simulink model "VehicleSilSimulation"  (R2026a)
settings: configuration reference "standardSILConfigurationParams" (kept outside this file)
StopFcn:
  | fid = fopen('C:\Users\Edison Altamirano\SITLV2\AnelloSummer\optimAeroPX4SIL\HILDiagnostics\logs\session_gtfix1\matlab_error_capture.txt','a'); fprintf(fid, '--- StopFcn fired at %s ---\n', datestr(now)); [m,i] = lasterr(); fprintf(fid, 'lasterr: %s (id: %s)\n', m, i); try; le = lasterror(); fprintf(fid, 'stack:\n'); for k=1:numel(le.stack); fprintf(fid, '  %s line %d\n', le.stack(k).name, le.stack(k).line); end; catch; end; fclose(fid);
values from neighbouring files (symbols this model uses):
  CONTROLLER_RUNTIME = 1    [initVehicleSIL.m]
  stepSize_s = 0.004    [initVehicleSIL.m]
  vehicleParams = evalin('base', 'vehicleParams')    [testVehicleSIL.m]
undefined symbols (not defined in the file or in its folder): actuatorDelay_s, controllerArmed, EngineCommandBus, gpsFreq, heartbeatFreq, opts, Payload, plantSampleTime_s, referenceLatitude_deg, referenceLongitude_deg, SampleTime, ServosCommandBus
libraries: uavmavlinklib x8, simulink x8, instrumentlib x6, flightGearInterfaceLibrary x6, aerolibfltsims x3, sharedtransform x3, px4MAVLinkBridgelib x2, aerolibanimutils x1, hdlsllib x1, dspnetwork x1, robotcorelib x1, uavutilslib x1
(part 1 of 3)
settings Model: SimulationMode=accelerator  Creator=GTAR  LastModifiedBy=Edison Altamirano
settings ConfigSetRef: SourceName=standardSILConfigurationParams  SourceLocation=Base Workspace

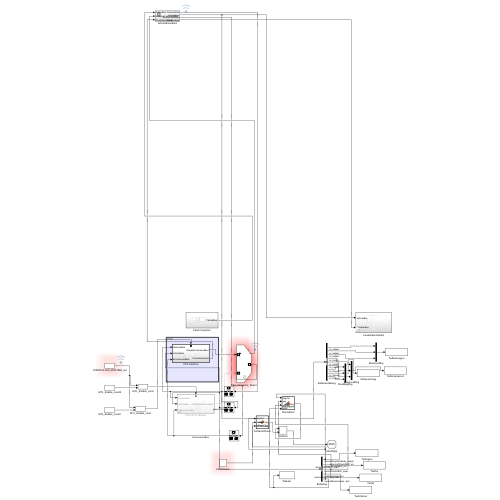
[thumbnail: Simulink's stored preview of the top-level diagram]
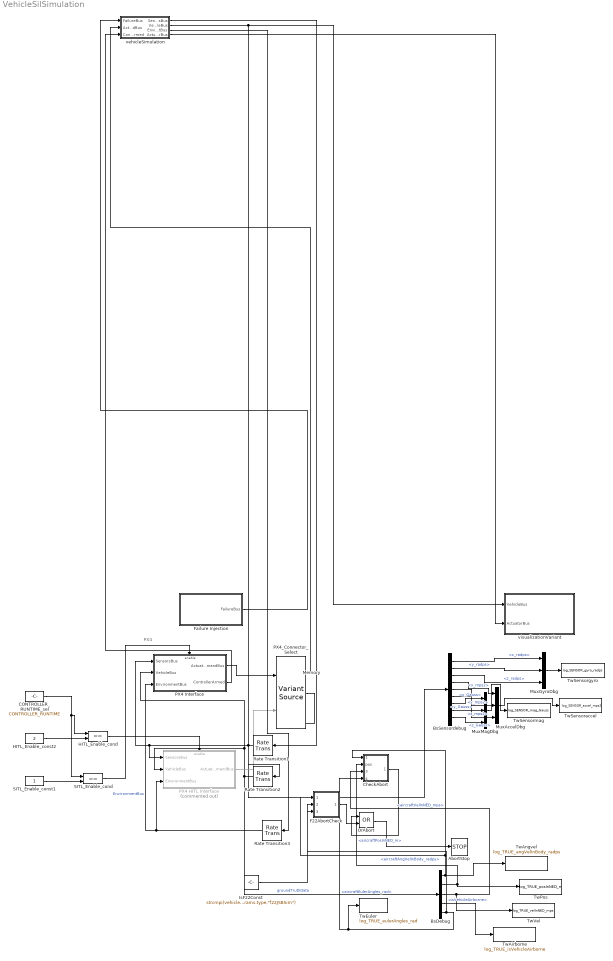
== system VehicleSilSimulation ==
  note: PX4
  AbortStop : Stop
  BsDebug : BusSelector  OutputSignals=signal2.aircraftAngVelInBody_radps,signal2.aircraftPosInNED_m,signal2.aircraftVelInNED_mps,signal1.isVehicleAirborne,signal2.aircraftEulerAngles_rad
  BsSensordebug : BusSelector  OutputSignals=INSSensorBus.GyroSensorBus.x_radps,INSSensorBus.GyroSensorBus.y_radps,INSSensorBus.GyroSensorBus.z_radps,INSSensorBus.AccelSensorBus.x_mps2,INSSensorBus.AccelSensorBus.y_mps2,INSSensorBus.AccelSensorBus.z_mps2,INSSensorBus.MagSensorBus.x_Gauss,INSSensorBus.MagSensorBus.y_Gauss,INSSensorBus.MagSensorBus.z_Gauss
  CONTROLLER_RUNTIME_sel : Constant  Value=CONTROLLER_RUNTIME
  CheckAbort : MATLAB Function  TreatAsAtomicUnit=on
  F22AbortCheck : MATLAB Function  TreatAsAtomicUnit=on
  Failure Injection : Subsystem
  HITL_Enable_cond : RelationalOperator  Operator===  OutDataTypeStr=boolean  RndMeth=Simplest  InputSameDT=off
  HITL_Enable_const2 : Constant  Value=2
  IsF22Const : Constant  Value="strcmpi(vehicleParams.type,\"f22JSBSim\")"
  Memory : Memory
  MuxAccelDbg : Mux  Inputs=3
  MuxGyroDbg : Mux  Inputs=3
  MuxMagDbg : Mux  Inputs=3
  OrAbort : Logic  Operator=OR
  PX4 HITL Interface : Subsystem  Commented=on
  PX4 Interface : Subsystem  VariantControl="strcmpi(vehicleParams.type, \"F-16\") & strcmpi(vehicleParams.controllerType, \"PX4\")"
  PX4_Connector_Select : VariantSource  VariantControls={CONTROLLER_RUNTIME == 1, CONTROLLER_RUNTIME == 2}
  Rate Transition1 : RateTransition
  Rate Transition2 : RateTransition
  Rate Transition3 : RateTransition
  SITL_Enable_cond : RelationalOperator  Operator===  OutDataTypeStr=boolean  RndMeth=Simplest  InputSameDT=off
  SITL_Enable_const1 : Constant
  TwAirborne : ToWorkspace  VariableName=log_TRUE_isVehicleAirborne  SaveFormat=Structure With Time  SampleTime=-1
  TwAngvel : ToWorkspace  VariableName=log_TRUE_angVelInBody_radps  SaveFormat=Structure With Time  SampleTime=-1
  TwEuler : ToWorkspace  VariableName=log_TRUE_eulerAngles_rad  SaveFormat=Timeseries  SampleTime=-1
  TwPos : ToWorkspace  VariableName=log_TRUE_posInNED_m  SaveFormat=Structure With Time  SampleTime=-1
  TwSensoraccel : ToWorkspace  VariableName=log_SENSOR_accel_mps2  SaveFormat=Structure With Time  SampleTime=-1
  TwSensorgyro : ToWorkspace  VariableName=log_SENSOR_gyro_radps  SaveFormat=Structure With Time  SampleTime=-1
  TwSensormag : ToWorkspace  VariableName=log_SENSOR_mag_Gauss  SaveFormat=Structure With Time  SampleTime=-1
  TwVel : ToWorkspace  VariableName=log_TRUE_velInNED_mps  SaveFormat=Structure With Time  SampleTime=-1
  vehicleSimulation : Subsystem
  visualizationVariant : Subsystem  Variant=on  EmptyChoice=on
  wires:
  Rate Transition1/1 -> PX4 Interface/1(SensorsBus), PX4 HITL Interface/1(SensorsBus), BsSensordebug/1
  Rate Transition2/1 -> PX4 HITL Interface/2(VehicleBus), PX4 Interface/2(VehicleBus), BsDebug/1  "groundTruthData"
  Rate Transition3/1 -> PX4 Interface/3(EnvironmentBus), PX4 HITL Interface/3(EnvironmentBus)  "EnvironmentBus"
  CONTROLLER_RUNTIME_sel/1 -> HITL_Enable_cond/1, SITL_Enable_cond/1
  HITL_Enable_const2/1 -> HITL_Enable_cond/2
  HITL_Enable_cond/1 -> PX4 HITL Interface/Enable
  SITL_Enable_const1/1 -> SITL_Enable_cond/2
  SITL_Enable_cond/1 -> PX4 Interface/Enable
  PX4 Interface/1(ActuatorCommandBus) -> PX4_Connector_Select/1
  PX4 HITL Interface/1(ActuatorCommandBus) -> PX4_Connector_Select/2
  PX4_Connector_Select/1 -> Memory/1
  BsDebug/1 -> F22AbortCheck/1(angVel), CheckAbort/1(angVel), TwAngvel/1  "<aircraftAngVelInBody_radps>"
  BsDebug/2 -> TwPos/1, CheckAbort/2(pos)  "<aircraftPosInNED_m>"
  BsDebug/3 -> TwVel/1, CheckAbort/3(velNED)  "<aircraftVelInNED_mps>"
  BsDebug/4 -> TwAirborne/1  "<isVehicleAirborne>"
  BsSensordebug/1 -> MuxGyroDbg/1  "<x_radps>"
  BsSensordebug/2 -> MuxGyroDbg/2  "<y_radps>"
  BsSensordebug/3 -> MuxGyroDbg/3  "<z_radps>"
  BsSensordebug/4 -> MuxAccelDbg/1  "<x_mps2>"
  BsSensordebug/5 -> MuxAccelDbg/2  "<y_mps2>"
  BsSensordebug/6 -> MuxAccelDbg/3  "<z_mps2>"
  MuxGyroDbg/1 -> TwSensorgyro/1
  MuxAccelDbg/1 -> TwSensoraccel/1
  BsDebug/5 -> TwEuler/1, CheckAbort/4(euler), F22AbortCheck/2(euler)  "<aircraftEulerAngles_rad>"
  BsSensordebug/7 -> MuxMagDbg/1  "<x_Gauss>"
  BsSensordebug/8 -> MuxMagDbg/2  "<y_Gauss>"
  BsSensordebug/9 -> MuxMagDbg/3  "<z_Gauss>"
  MuxMagDbg/1 -> TwSensormag/1
  CheckAbort/1(abortFlag) -> OrAbort/1
  F22AbortCheck/1(abortFlag) -> OrAbort/2
  OrAbort/1 -> AbortStop/1
  IsF22Const/1 -> F22AbortCheck/3(isF22Active)
  vehicleSimulation/1(SensorsBus) -> Rate Transition1/1
  vehicleSimulation/2(VehicleBus) -> Rate Transition2/1, visualizationVariant/1(VehicleBus)
  vehicleSimulation/3(EnvironmentBus) -> Rate Transition3/1
  vehicleSimulation/4(ActuatorBus) -> visualizationVariant/2(ActuatorBus)
  Failure Injection/1(FailureBus) -> vehicleSimulation/1(FailureBus)
  Memory/1 -> vehicleSimulation/2(ActuatorCommandBus)
  PX4 Interface/2(ControllerArmed) -> vehicleSimulation/3(ControllerArmed)

== system VehicleSilSimulation/Failure Injection ==
  Constant : Constant  Value=vehicleParams.failureType
  PilotJoystick : aerolibanimutils/Pilot Joystick  JoystickID=None  OutputConfiguration=AllOutputs  SampleTime=stepSize_s
      settings: LibrarySourceBlock=aerolibanimutils/Pilot Joystick All
  Variant Model : Subsystem  Variant=on
  FailureBus : Outport
  wires:
  PilotJoystick/2 -> Variant Model/2(buttons)
  Variant Model/1(FailureBus) -> FailureBus/1
  PilotJoystick/3 -> Variant Model/3(POV)
  PilotJoystick/1 -> Variant Model/1(analog)
  Constant/1 -> Variant Model/4(failureType)

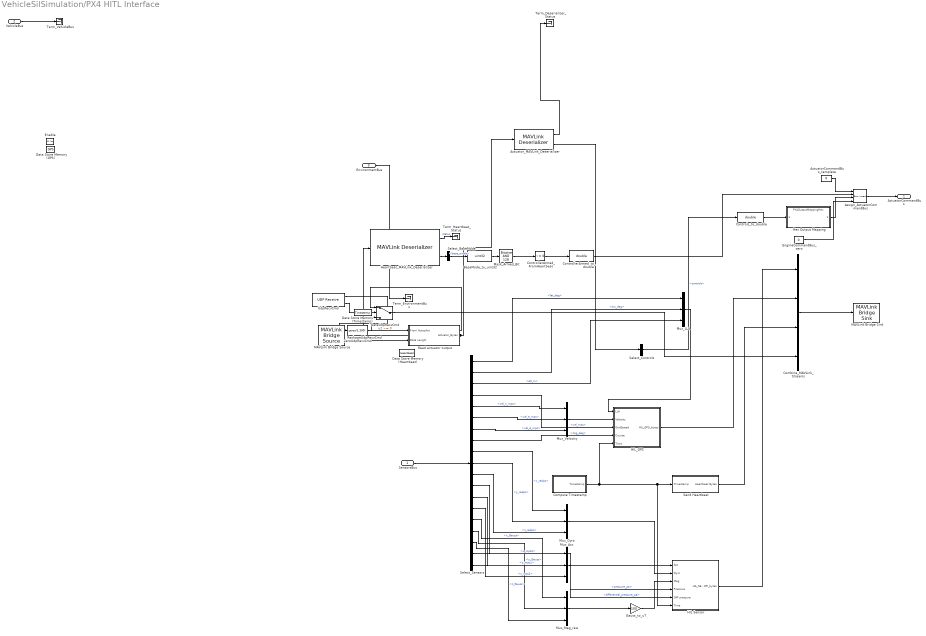
== system VehicleSilSimulation/PX4 HITL Interface ==
  SensorsBus : Inport  OutDataTypeStr=Bus: SensorsBus
  VehicleBus : Inport  Port=2  OutDataTypeStr=Bus: VehicleBus
  EnvironmentBus : Inport  Port=3  OutDataTypeStr=Bus: EnvironmentBus
  Enable : EnablePort  PropagateVarSize=During execution
  ActuatorCommandBus_template : Constant  Value=0  OutDataTypeStr=Bus: ActuatorCommandBus
  Actuator_MAVLink_Deserializer : uavmavlinklib/MAVLink Deserializer  dialectSource=Select from standard MAVLink dialects  dialect=common.xml  dialectCustom=common.xml  version=2  messageType=HIL_ACTUATOR_CONTROLS  inputDataLength=off  SystemIDFilter=off  systemID=1  ComponentIDFilter=off  componentID=1  queueMsg=off  queueMsgSize=50  dropNum=off
  Assign_ActuatorCommandBus : BusAssignment  AssignedSignals=controllerArmed,ServosCommandBus,EngineCommandBus
  BaseMode_to_uint32 : DataTypeConversion  OutDataTypeStr=uint32
  Combine_MAVLink_Streams : Mux
  Compute Timestamp : Subsystem  Priority=1
  ControllerArmed_FromHeartbeat : hdlsllib/Logic and Bit Operations/Compare To Zero  relop=~=  OutDataTypeStr=uint8
  ControllerArmed_to_double : DataTypeConversion  OutDataTypeStr=double
  Controls_to_double : DataTypeConversion  OutDataTypeStr=double  SaturateOnIntegerOverflow=off  RndMeth=Floor
  Data Store Memory (GPS) : DataStoreMemory  DataStoreName=GPS  WriteAfterWriteMsg=warning  ShowAdditionalParam=off
  Data Store Memory (Heartbeat) : DataStoreMemory  DataStoreName=Heartbeat  WriteAfterWriteMsg=warning  ShowAdditionalParam=off
  Data Store Memory (Timestamp) : DataStoreMemory  DataStoreName=Timestamp  WriteAfterWriteMsg=warning  ShowAdditionalParam=off
  EngineCommandBus_zero : Constant  Value=0  OutDataTypeStr=Bus: EngineCommandBus
  GateUdpRecvCmd : Switch  Criteria=u2 ~= 0  SaturateOnIntegerOverflow=off  InputSameDT=off
  Gauss_to_uT : Gain  Gain=100
  HIL Sensor : Subsystem  Priority=2
  HIL_GPS : Subsystem  Priority=3
  Heartbeat_MAVLink_Deserializer : uavmavlinklib/MAVLink Deserializer  dialectSource=Select from standard MAVLink dialects  dialect=common.xml  dialectCustom=common.xml  version=2  messageType=HEARTBEAT  inputDataLength=off  SystemIDFilter=off  systemID=1  ComponentIDFilter=off  componentID=1  queueMsg=off  queueMsgSize=50  dropNum=off
  Hex Output Mapping : ModelReference  ModelNameDialog=PX4OutputMappingHex.slx  SimulationMode=Normal  ModelReferenceVersion=1.15
  MAVLink Bridge Sink : px4MAVLinkBridgelib/MAVLink Bridge Sink  PixhawkSerialPorttemp=Specify manually  PixhawkSerialPortManually=COM4  FieldTable={'UDP', '127.0.0.1', '14550'}
  MAVLink Bridge Source : px4MAVLinkBridgelib/MAVLink Bridge Source  PixhawkSerialPorttemp=Specify manually  PixhawkSerialPortManually=COM4  dataLength=1024  FieldTable={'UDP', '127.0.0.1', '14550'}  SampleTime=SampleTime
  Mask_Armed_Bit : simulink/Logic and Bit Operations/Bitwise Operator  logicop=AND  UseBitMask=on  BitMask=128  BitMaskRealWorld=Stored Integer
      settings: LibrarySourceBlock=|
      | hdlsllib/Logic and Bit
      | Operations/Bitwise
      | Operator
  Mux_Acc : Mux  Inputs=3
  Mux_Gyro : Mux  Inputs=3
  Mux_LLA : Mux  Inputs=3
  Mux_Mag_raw : Mux  Inputs=3
  Mux_Velocity : Mux  Inputs=3
  Read actuator output : Subsystem
  ReshapeUdpRecvCmd : Reshape
  Select_BaseMode : BusSelector  OutputSignals=Payload.base_mode
  Select_Controls : BusSelector  OutputSignals=Payload.controls
  Select_Sensors : BusSelector  OutputSignals=GPSSensorBus.lat_deg,GPSSensorBus.lon_deg,GPSSensorBus.alt_m,GPSSensorBus.vel_mps,GPSSensorBus.vel_n_mps,GPSSensorBus.vel_e_mps,GPSSensorBus.vel_d_mps,GPSSensorBus.cog_deg,INSSensorBus.GyroSensorBus.x_radps,INSSensorBus.GyroSensorBus.y_radps,INSSensorBus.GyroSensorBus.z_radps,INSSensorBus.AccelSensorBus.x_mps2,INSSensorBus.AccelSensorBus.y_mps2,INSSensorBus.AccelSensorBus.z_mps2,INSSensorBus.MagSensorBus.x_Gauss,INSSensorBus.MagSensorBus.y_Gauss,INSSensorBus.MagSensorBus.z_Gauss,ADCSensorBus.BaroSensorBus.pressure_pa,ADCSensorBus.DiffPressureSensorBus.differential_pressure_pa
  Send Heartbeat : Subsystem  Priority=4
  Term_Deserializer_Status : Terminator
  Term_EnvironmentBus : Terminator
  Term_Heartbeat_Status : Terminator
  Term_VehicleBus : Terminator
  UdpRecvCmd : dspnetwork/UDP Receive  localURL='0.0.0.0'  localPort=14541  remoteURL='0.0.0.0'  remotePort=-1  recvBufferSize=8192  dims=300  signalDatatype=uint8  isComplex=off  isVarSize=off  showBlockingTime=off  blockingTime=0  sampletime=SampleTime  blockPlatform=[]
      settings: LibrarySourceBlock=dspsrcs4/UDP Receive
  ZeroUdpRecvCmd : Constant  Value=zeros(1,300)  OutDataTypeStr=uint8
  ActuatorCommandBus : Outport  OutDataTypeStr=Bus: ActuatorCommandBus
  wires:
  Select_Sensors/18 -> HIL Sensor/4(Pressure)  "<pressure_pa>"
  Select_Sensors/1 -> Mux_LLA/1  "<lat_deg>"
  HIL_GPS/1(HIL_GPS_bytes) -> Combine_MAVLink_Streams/2
  Actuator_MAVLink_Deserializer/1 -> Term_Deserializer_Status/1
  VehicleBus/1 -> Term_VehicleBus/1
  MAVLink Bridge Source/2 -> Read actuator output/2(Data Length)
  Read actuator output/1(Actuator_Bytes) -> Actuator_MAVLink_Deserializer/1, Heartbeat_MAVLink_Deserializer/1
  Mux_Mag_raw/1 -> Gauss_to_uT/1
  SensorsBus/1 -> Select_Sensors/1
  EnvironmentBus/1 -> Term_EnvironmentBus/1
  MAVLink Bridge Source/1 -> Read actuator output/1(From Autopilot)
  Select_Sensors/2 -> Mux_LLA/2  "<lon_deg>"
  Mux_Acc/1 -> HIL Sensor/1(Acc)
  Select_Sensors/3 -> Mux_LLA/3  "<alt_m>"
  Mux_Gyro/1 -> HIL Sensor/2(Gyro)
  Actuator_MAVLink_Deserializer/2 -> Select_Controls/1
  Select_Sensors/4 -> HIL_GPS/3(GndSpeed)  "<vel_mps>"
  Select_Sensors/5 -> Mux_Velocity/1  "<vel_n_mps>"
  Select_Sensors/11 -> Mux_Gyro/3  "<z_radps>"
  Select_Sensors/6 -> Mux_Velocity/2  "<vel_e_mps>"
  Select_Sensors/7 -> Mux_Velocity/3  "<vel_d_mps>"
  Mux_Velocity/1 -> HIL_GPS/2(Velocity)
  Select_Sensors/8 -> HIL_GPS/4(Course)  "<cog_deg>"
  HIL Sensor/1(HIL_SENSOR_bytes) -> Combine_MAVLink_Streams/1
  Select_Sensors/9 -> Mux_Gyro/1  "<x_radps>"
  ActuatorCommandBus_template/1 -> Assign_ActuatorCommandBus/1
  Select_Sensors/10 -> Mux_Gyro/2  "<y_radps>"
  Select_Sensors/12 -> Mux_Acc/1  "<x_mps2>"
  Select_Sensors/13 -> Mux_Acc/2  "<y_mps2>"
  Select_Sensors/14 -> Mux_Acc/3  "<z_mps2>"
  Select_Sensors/15 -> Mux_Mag_raw/1  "<x_Gauss>"
  Select_Sensors/16 -> Mux_Mag_raw/2  "<y_Gauss>"
  Select_Sensors/17 -> Mux_Mag_raw/3  "<z_Gauss>"
  Select_Sensors/19 -> HIL Sensor/5(Diff pressure)  "<differential_pressure_pa>"
  Mux_LLA/1 -> HIL_GPS/1(LLA)
  Compute Timestamp/1(Timestamp) -> HIL Sensor/6(Time), Send Heartbeat/1(Timestamp), HIL_GPS/5(Time)
  Controls_to_double/1 -> Hex Output Mapping/1
  Select_Controls/1 -> Controls_to_double/1  "<controls>"
  Gauss_to_uT/1 -> HIL Sensor/3(Mag)
  Combine_MAVLink_Streams/1 -> MAVLink Bridge Sink/1
  Send Heartbeat/1(Heartbeat Bytes) -> Combine_MAVLink_Streams/3
  Hex Output Mapping/1 -> Assign_ActuatorCommandBus/3
  EngineCommandBus_zero/1 -> Assign_ActuatorCommandBus/4
  Assign_ActuatorCommandBus/1 -> ActuatorCommandBus/1
  Heartbeat_MAVLink_Deserializer/1 -> Term_Heartbeat_Status/1  "status"
  Heartbeat_MAVLink_Deserializer/2 -> Select_BaseMode/1
  Select_BaseMode/1 -> BaseMode_to_uint32/1  "<base_mode>"
  BaseMode_to_uint32/1 -> Mask_Armed_Bit/1
  Mask_Armed_Bit/1 -> ControllerArmed_FromHeartbeat/1
  ControllerArmed_FromHeartbeat/1 -> ControllerArmed_to_double/1
  ControllerArmed_to_double/1 -> Assign_ActuatorCommandBus/2
  UdpRecvCmd/1 -> ReshapeUdpRecvCmd/1
  ReshapeUdpRecvCmd/1 -> GateUdpRecvCmd/1
  UdpRecvCmd/2 -> GateUdpRecvCmd/2
  ZeroUdpRecvCmd/1 -> GateUdpRecvCmd/3
  GateUdpRecvCmd/1 -> Combine_MAVLink_Streams/4

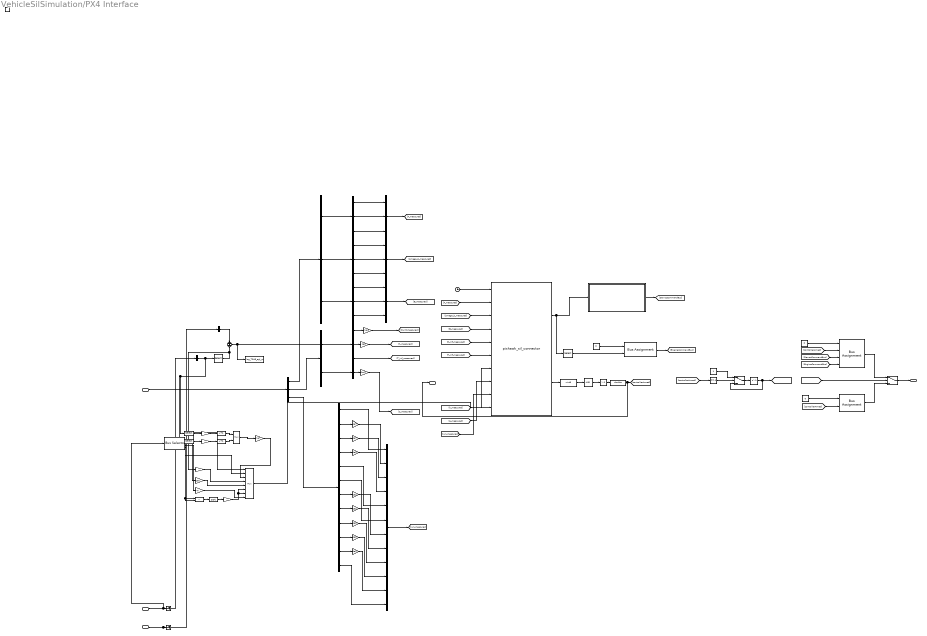
== system VehicleSilSimulation/PX4 Interface ==
  note: TODO: Signals that will be used for truth data
  note: TODO: Investigate use of truth data
  note: https://fst.aviumtechnologies.com/pixhawk-sil-connector
  note: Sil Connector designed by:
  note: sil_connector uses time since start in [s]
  SensorsBus : Inport  OutDataTypeStr=Bus: SensorsBus
  VehicleBus : Inport  Port=2  OutDataTypeStr=Bus: VehicleBus
  EnvironmentBus : Inport  Port=3  OutDataTypeStr=Bus: EnvironmentBus
  Enable : EnablePort  PropagateVarSize=During execution
  AglCompute : Sum  Inputs=+-
  AglPosZSel : Selector  InputPortWidth=3  IndexOptions=Index vector (dialog)  Indices=3  OutputSizes=1
  AglTerrainSel : BusSelector  OutputSignals=TerrainEnvironment.terrainHeightInNED_m
  AglVehicleSel : BusSelector  OutputSignals=signal2.aircraftPosInNED_m
  Bitwise Operator : simulink/Logic and Bit Operations/Bitwise Operator  logicop=AND  UseBitMask=on  BitMask=bin2dec('10000000')  BitMaskRealWorld=Stored Integer
  Bus Assignment1 : BusAssignment  AssignedSignals=cmdThrottle_unit
  Bus Assignment2 : BusAssignment  AssignedSignals=controllerArmed
  Bus Assignment3 : BusAssignment  AssignedSignals=controllerArmed,ServosCommandBus,EngineCommandBus
  Bus Selector : BusSelector  OutputSignals=INSSensorBus,ADCSensorBus,GPSSensorBus
  Bus Selector1 : BusSelector  OutputSignals=AccelSensorBus,GyroSensorBus,MagSensorBus
  Bus Selector2 : BusSelector  OutputSignals=BaroSensorBus,DiffPressureSensorBus
  Bus Selector3 : BusSelector  OutputSignals=device_id,lat_deg,lon_deg,alt_m,eph_m,epv_m,vel_mps,vel_n_mps,vel_e_mps,vel_d_mps,cog_deg,satellites_used_nd
  Bus Selector4 : BusSelector  OutputSignals=x_mps2,y_mps2,z_mps2
  Bus Selector5 : BusSelector  OutputSignals=x_radps,y_radps,z_radps
  Bus Selector6 : BusSelector  OutputSignals=pressure_pa,altitude_m,temperature_degC
  Bus Selector7 : BusSelector  OutputSignals=differential_pressure_pa
  Bus Selector8 : BusSelector  OutputSignals=x_Gauss,y_Gauss,z_Gauss
  Clock : Clock
  Command Output Variaint : Subsystem  Variant=on
  Compare To Zero : simulink/Logic and Bit Operations/Compare To Zero  relop=>  OutDataTypeStr=uint8
  Compare To Zero1 : simulink/Logic and Bit Operations/Compare To Zero  relop===  OutDataTypeStr=boolean
  Constant : Constant
  Constant1 : Constant  Value=0  OutDataTypeStr=Bus: ActuatorCommandBus
  Constant3 : Constant  Value=0  OutDataTypeStr=Bus: ActuatorCommandBus
  Data Type Conversion2 : DataTypeConversion  OutDataTypeStr=uint8  SaturateOnIntegerOverflow=off  RndMeth=Floor
  Data Type Conversion3 : DataTypeConversion  OutDataTypeStr=double  SaturateOnIntegerOverflow=off  RndMeth=Floor
  Delay : Delay  DelayLength=1  InitialCondition=0
  EngineCommandBus : Constant  Value=0  OutDataTypeStr=Bus: EngineCommandBus
  GTAccelGain : Gain  Gain=101.9716
  GTAltGain : Gain  Gain=-1000
  GTAsDot : DotProduct  OutDataTypeStr=Inherit: Inherit via internal rule
  GTAsGain : Gain  Gain=100
  GTAsSqrt : Math  Operator=sqrt
  GTBusSel : BusSelector  OutputSignals=signal2.aircraftEulerAngles_rad,signal2.aircraftAngVelInBody_radps,signal2.aircraftVelInNED_mps,signal2.aircraftAccelbe_mps2,signal5.airspeedInBody_mps
  GTEastSel : Selector  InputPortWidth=3  IndexOptions=Index vector (dialog)  Indices=[2]  OutputSizes=1
  GTFinalMux : Mux  Inputs=8
  GTLatBias : Bias  Bias=referenceLatitude_deg  SaturateOnIntegerOverflow=off
  GTLatGain : Gain  Gain=180/(pi*6378137)
  GTLatLonGain : Gain  Gain=1e7
  GTLatLonMux2 : Mux  Inputs=2
  GTLonBias : Bias  Bias=referenceLongitude_deg  SaturateOnIntegerOverflow=off
  GTLonGain : Gain  Gain=180/(pi*6378137*cosd(referenceLatitude_deg))
  GTNorthSel : Selector  InputPortWidth=3  IndexOptions=Index vector (dialog)  Indices=[1]  OutputSizes=1
  GTVelGain : Gain  Gain=100
  Gain : Gain  Gain=1e-2
  Gain1 : Gain  Gain=1e3
  Gain11 : Gain  Gain=1e-2
  Gain{2..7} (6 alike) : Gain  Gain=1e2
  Gain8 : Gain  Gain=1e7
  Gain9 : Gain  Gain=1e7
  Mux : Mux  Inputs=3
  Mux1 : Mux  Inputs=3
  Mux2 : Mux  Inputs=3
  Mux3 : Mux  Inputs=12
  S-Function : S-Function  FunctionName=pixhawk_sil_connector  SFunctionDeploymentMode=off  EnableBusSupport=off
  Selector : Selector  InputPortWidth=16  IndexOptions=Index vector (dialog)  Indices=[1]  OutputSizes=1
  Switch7 : Switch  Criteria=u2 > Threshold  SaturateOnIntegerOverflow=off  InputSameDT=off
  Switch8 : Switch  Criteria=u2 > Threshold  SaturateOnIntegerOverflow=off  InputSameDT=off
  Terminator : Terminator
  Terminator1 : Terminator
  TwAgl : ToWorkspace  VariableName=log_TRUE_agl_m  SaveFormat=Structure With Time  SampleTime=-1
  ActuatorCommandBus : Outport  OutDataTypeStr=Bus: ActuatorCommandBus  LockScale=on
  ControllerArmed : Outport  Port=2
  wires:
  Bus Selector7/1 -> Gain11/1  "<differential_pressure_pa>"
  Bus Selector4/3 -> Mux/3  "<z_mps2>"
  Bus Selector4/2 -> Mux/2  "<y_mps2>"
  Bus Selector4/1 -> Mux/1  "<x_mps2>"
  Bus Selector5/2 -> Mux1/2  "<y_radps>"
  Bus Selector6/1 -> Gain/1  "<pressure_pa>"
  Bus Selector5/1 -> Mux1/1  "<x_radps>"
  Bus Selector5/3 -> Mux1/3  "<z_radps>"
  Bus Selector3/7 -> Gain2/1  "<vel_mps>"
  Bus Selector3/5 -> Mux3/5  "<eph_m>"
  Bus Selector3/4 -> Gain1/1  "<alt_m>"
  Bus Selector3/3 -> Gain9/1  "<lon_deg>"
  Bus Selector3/2 -> Gain8/1  "<lat_deg>"
  Bus Selector2/2 -> Bus Selector7/1  "<DiffPressureSensorBus>"
  Bus Selector2/1 -> Bus Selector6/1  "<BaroSensorBus>"
  Bus Selector/2 -> Bus Selector2/1  "<ADCSensorBus>"
  Bus Selector1/2 -> Bus Selector5/1  "<GyroSensorBus>"
  Bus Selector/1 -> Bus Selector1/1  "<INSSensorBus>"
  Bus Selector/3 -> Bus Selector3/1  "<GPSSensorBus>"
  SensorsBus/1 -> Bus Selector/1
  Bus Selector1/1 -> Bus Selector4/1  "<AccelSensorBus>"
  Bus Selector1/3 -> Bus Selector8/1  "<MagSensorBus>"
  Bus Selector8/1 -> Mux2/1  "<x_Gauss>"
  Bus Selector8/2 -> Mux2/2  "<y_Gauss>"
  Bus Selector8/3 -> Mux2/3  "<z_Gauss>"
  Clock/1 -> S-Function/1  "time_s"
  Selector/1 -> Bus Assignment1/2
  S-Function/1 -> Command Output Variaint/1(PX4 Output Commands), Selector/1
  S-Function/2 -> Data Type Conversion2/1
  Data Type Conversion2/1 -> Bitwise Operator/1
  Bitwise Operator/1 -> Compare To Zero/1
  Compare To Zero/1 -> Data Type Conversion3/1
  Data Type Conversion3/1 -> ControllerArmed/1, [controllerArmed]
  Switch7/1 -> ActuatorCommandBus/1
  Switch8/1 -> Delay/1
  [controllerArmed] -> Compare To Zero1/1
  Constant/1 -> Switch8/1
  Compare To Zero1/1 -> Switch8/2
  Delay/1 -> Switch8/3, [controllerInitialized]
  [controllerInitialized] -> Switch7/2
  EngineCommandBus/1 -> Bus Assignment1/1
  Bus Assignment1/1 -> [EngineCommandBus]
  [controllerArmed] -> Bus Assignment2/2
  Constant3/1 -> Bus Assignment2/1
  Bus Assignment2/1 -> Switch7/3
  Constant1/1 -> Bus Assignment3/1
  [ServosCommandBus] -> Bus Assignment3/3
  [EngineCommandBus] -> Bus Assignment3/4
  [controllerArmed] -> Bus Assignment3/2
  Bus Assignment3/1 -> Switch7/1
  VehicleBus/1 -> GTBusSel/1, AglVehicleSel/1, Terminator/1
  EnvironmentBus/1 -> AglTerrainSel/1, Terminator1/1
  [omega_b_measured] -> S-Function/3
  [B_measured] -> S-Function/4
  [P_inf_measured] -> S-Function/5
  [T_inf_measured] -> S-Function/6
  [q_measured] -> S-Function/8
  [h_measured] -> S-Function/7
  Bus Selector3/1 -> Mux3/1  "<device_id>"
  Gain1/1 -> Mux3/4
  Bus Selector3/6 -> Mux3/6  "<epv_m>"
  Gain2/1 -> Mux3/7
  Bus Selector3/8 -> Gain3/1  "<vel_n_mps>"
  Bus Selector3/9 -> Gain4/1  "<vel_e_mps>"
  Bus Selector3/10 -> Gain5/1  "<vel_d_mps>"
  Bus Selector3/11 -> Gain6/1  "<cog_deg>"
  Bus Selector3/12 -> Mux3/12  "<satellites_used_nd>"
  Gain3/1 -> Mux3/8
  Gain4/1 -> Mux3/9
  Gain5/1 -> Mux3/10
  Gain6/1 -> Mux3/11
  [xyz_measured] -> S-Function/9
  Mux3/1 -> [xyz_measured]  "xyz_optim"
  Gain/1 -> [P_inf_measured]  "baro_hPa"
  Gain7/1 -> [h_measured]
  Bus Selector6/3 -> [T_inf_measured]  "<temperature_degC>"
  Gain11/1 -> [q_measured]  "dyn_press_hPa"
  Mux2/1 -> [B_measured]  "mag_gauss"
  Mux1/1 -> [omega_b_measured]
  Mux/1 -> [A_measured]  "accel_mps2"
  Gain8/1 -> Mux3/2
  Gain9/1 -> Mux3/3
  [A_measured] -> S-Function/2
  Command Output Variaint/1(ServosCommandBusOut) -> [ServosCommandBus]
  AglVehicleSel/1 -> GTEastSel/1, GTNorthSel/1, AglPosZSel/1  "<aircraftPosInNED_m>"
  AglTerrainSel/1 -> AglCompute/1  "<terrainHeightInNED_m>"
  AglPosZSel/1 -> GTAltGain/1, AglCompute/2
  AglCompute/1 -> Gain7/1, TwAgl/1
  GTBusSel/3 -> GTVelGain/1  "<aircraftVelInNED_mps>"
  GTBusSel/4 -> GTAccelGain/1  "<aircraftAccelbe_mps2>"
  GTBusSel/5 -> GTAsDot/2, GTAsDot/1  "<airspeedInBody_mps>"
  GTAsDot/1 -> GTAsSqrt/1
  GTAsSqrt/1 -> GTAsGain/1
  GTBusSel/1 -> GTFinalMux/1  "<aircraftEulerAngles_rad>"
  GTBusSel/2 -> GTFinalMux/2  "<aircraftAngVelInBody_radps>"
  GTLatLonGain/1 -> GTFinalMux/3
  GTAltGain/1 -> GTFinalMux/4
  GTVelGain/1 -> GTFinalMux/5
  GTAsGain/1 -> GTFinalMux/7, GTFinalMux/6
  GTAccelGain/1 -> GTFinalMux/8
  GTFinalMux/1 -> S-Function/10
  GTNorthSel/1 -> GTLatGain/1
  GTLatGain/1 -> GTLatBias/1
  GTEastSel/1 -> GTLonGain/1
  GTLonGain/1 -> GTLonBias/1
  GTLatBias/1 -> GTLatLonMux2/1
  GTLonBias/1 -> GTLatLonMux2/2
  GTLatLonMux2/1 -> GTLatLonGain/1

== system VehicleSilSimulation/vehicleSimulation ==
  note: from PX4
  FailureBus : Inport  OutDataTypeStr=Bus: FailureBus
  ActuatorCommandBus : Inport  Port=2  OutDataTypeStr=Bus: ActuatorCommandBus  LockScale=on
  ControllerArmed : Inport  Port=3
  Memory : Memory
  environment : ModelReference  ModelNameDialog=environment.slx  SimulationMode=Normal  ModelReferenceVersion=1.14
  plant : Subsystem  Variant=on
  sensors : ModelReference  ModelNameDialog=sensors.slx  SimulationMode=Normal  ModelReferenceVersion=5.1
  SensorsBus : Outport  OutDataTypeStr=Bus: SensorsBus
  VehicleBus : Outport  Port=2  OutDataTypeStr=Bus: VehicleBus
  EnvironmentBus : Outport  Port=3  OutDataTypeStr=Bus: EnvironmentBus
  ActuatorBus : Outport  Port=4  OutDataTypeStr=Bus: ActuatorBus
  wires:
  sensors/1 -> SensorsBus/1
  ActuatorCommandBus/1 -> plant/1(ActuatorCommandBus)
  environment/1 -> sensors/1, EnvironmentBus/1, plant/2(EnvironmentBus)
  Memory/1 -> environment/1, sensors/2
  plant/1(VehicleBus) -> Memory/1, VehicleBus/1
  FailureBus/1 -> [FailureBus]
  [FailureBus] -> plant/3(FailureBus)
  plant/2(ActuatorBus) -> ActuatorBus/1
  ControllerArmed/1 -> plant/4(ControllerArmed)

== system VehicleSilSimulation/visualizationVariant ==
  note: 1) Add Subsystem or Model blocks as valid variant choices.
      | 2) You cannot connect blocks at this level. At simulation, connectivity is automatically
      | determined, based on the active variant and port name matching.
  VehicleBus : Inport
  ActuatorBus : Inport  Port=2
  FlightGearVisualizationF16 : Subsystem  TreatAsAtomicUnit=on  VariantControl="strcmpi(opts.visualizationType, \"FlightGear\") && strcmpi (vehicleParams.type, \"F-16\")"
  FlightGearVisualizationFixedWing : Subsystem  TreatAsAtomicUnit=on  VariantControl="strcmpi(opts.visualizationType, \"FlightGear\") && (strcmpi(vehicleParams.type,\"c172p\") || strcmpi(vehicleParams.type,\"c172pJSBSim\") || strcmpi(vehicleParams.type,\"c130JSBSim\") || strcmpi(vehicleParams.type,\"f22JSBSim\"))"
  FlightGearVisualizationHexarotor : Subsystem  TreatAsAtomicUnit=on  VariantControl="strcmpi(opts.visualizationType, \"FlightGear\") && strcmpi (vehicleParams.type, \"hexarotor\")"
  MatlabVisualization : Subsystem  VariantControl="strcmpi(opts.visualizationType, \"Matlab\")"
  passthrough : Subsystem  VariantControl="strcmpi(opts.visualizationType, \"PassThrough\")"

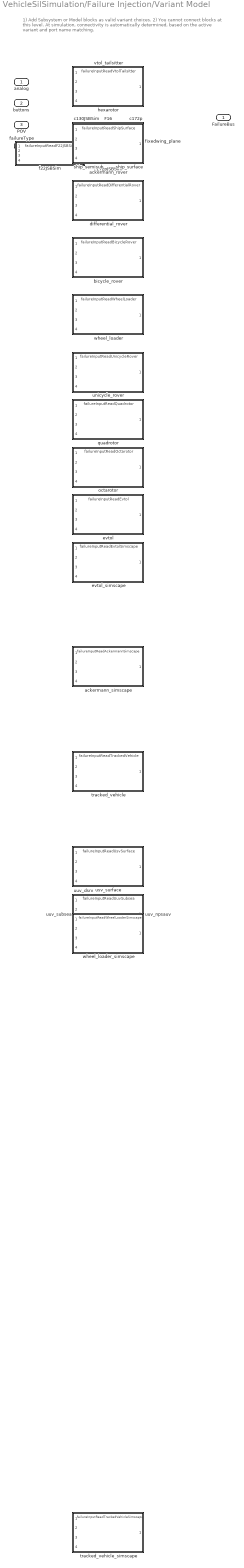
== system VehicleSilSimulation/Failure Injection/Variant Model ==
  note: 1) Add Subsystem or Model blocks as valid variant choices.
      | 2) You cannot connect blocks at this level. At simulation, connectivity is automatically
      | determined, based on the active variant and port name matching.
  analog : Inport
  buttons : Inport  Port=2
  POV : Inport  Port=3
  failureType : Inport  Port=4
  F16 : ModelReference  ModelNameDialog=failureInputReadF16.slx  VariantControl="strcmpi(vehicleParams.type, \"F16\")"  ModelReferenceVersion=1.18
  ackermann_rover : ModelReference  ModelNameDialog=failureInputReadAckermannRover.slx  SimulationMode=Normal  VariantControl="strcmpi(vehicleParams.type, \"ackermann_rover\")"  ModelReferenceVersion=1.6
  ackermann_simscape : ModelReference  ModelNameDialog=failureInputReadAckermannSimscape.slx  SimulationMode=Normal  VariantControl="strcmpi(vehicleParams.type, \"ackermann_simscape\")"  ModelReferenceVersion=1.6
  bicycle_rover : ModelReference  ModelNameDialog=failureInputReadBicycleRover.slx  SimulationMode=Normal  VariantControl="strcmpi(vehicleParams.type, \"bicycle_rover\")"  ModelReferenceVersion=1.1
  c130JSBSim : ModelReference  ModelNameDialog=failureInputReadC130JSBSim  VariantControl="strcmpi(vehicleParams.type, \"c130JSBSim\")"  ModelReferenceVersion=1.18
  c172p : ModelReference  ModelNameDialog=failureInputReadC172p  VariantControl="strcmpi(vehicleParams.type, \"c172p\")"  ModelReferenceVersion=1.18
  c172pJSBSim : ModelReference  ModelNameDialog=failureInputReadC172pJSBSim.slx  VariantControl="strcmpi(vehicleParams.type, \"c172pJSBSim\")"  ModelReferenceVersion=1.18
  differential_rover : ModelReference  ModelNameDialog=failureInputReadDifferentialRover.slx  SimulationMode=Normal  VariantControl="strcmpi(vehicleParams.type, \"differential_rover\")"  ModelReferenceVersion=1.1
  evtol : ModelReference  ModelNameDialog=failureInputReadEvtol.slx  SimulationMode=Normal  VariantControl="strcmpi(vehicleParams.type, \"evtol\")"  ModelReferenceVersion=5.0
  evtol_simscape : ModelReference  ModelNameDialog=failureInputReadEvtolSimscape.slx  SimulationMode=Normal  VariantControl="strcmpi(vehicleParams.type, \"evtol_simscape\")"  ModelReferenceVersion=5.0
  f22JSBSim : ModelReference  ModelNameDialog=failureInputReadF22JSBSim  SimulationMode=Normal  VariantControl="strcmpi(vehicleParams.type, \"f22JSBSim\")"  ModelReferenceVersion=1.18
  fixedwing_plane : ModelReference  ModelNameDialog=failureInputReadFixedwingPlane.slx  VariantControl="strcmpi(vehicleParams.type, \"fixedwing_plane\")"  ModelReferenceVersion=1.18
  hexarotor : ModelReference  DisableCoverage=on  ModelNameDialog=failureInputReadHex.slx  VariantControl="strcmpi(vehicleParams.type, \"hexarotor\")"  ModelReferenceVersion=1.56
  octarotor : ModelReference  ModelNameDialog=failureInputReadOctarotor.slx  SimulationMode=Normal  VariantControl="strcmpi(vehicleParams.type, \"octarotor\")"  ModelReferenceVersion=1.1
  quadrotor : ModelReference  ModelNameDialog=failureInputReadQuadrotor.slx  SimulationMode=Normal  VariantControl="strcmpi(vehicleParams.type, \"quadrotor\")"  ModelReferenceVersion=1.1
  ship_semisub : ModelReference  ModelNameDialog=failureInputReadShipSemisub.slx  SimulationMode=Normal  VariantControl="strcmpi(vehicleParams.type, \"ship_semisub\")"  ModelReferenceVersion=1.6
  ship_surface : ModelReference  ModelNameDialog=failureInputReadShipSurface.slx  SimulationMode=Normal  VariantControl="strcmpi(vehicleParams.type, \"ship_surface\")"  ModelReferenceVersion=1.6
  tracked_vehicle : ModelReference  ModelNameDialog=failureInputReadTrackedVehicle.slx  SimulationMode=Normal  VariantControl="strcmpi(vehicleParams.type, \"tracked_vehicle\")"  ModelReferenceVersion=1.1
  tracked_vehicle_simscape : ModelReference  ModelNameDialog=failureInputReadTrackedVehicleSimscape.slx  SimulationMode=Normal  VariantControl="strcmpi(vehicleParams.type, \"tracked_vehicle_simscape\")"  ModelReferenceVersion=1.1
  unicycle_rover : ModelReference  ModelNameDialog=failureInputReadUnicycleRover.slx  SimulationMode=Normal  VariantControl="strcmpi(vehicleParams.type, \"unicycle_rover\")"  ModelReferenceVersion=1.1
  usv_surface : ModelReference  ModelNameDialog=failureInputReadUsvSurface.slx  SimulationMode=Normal  VariantControl="strcmpi(vehicleParams.type, \"usv_surface\")"  ModelReferenceVersion=1.1
  uuv_dsrv : ModelReference  ModelNameDialog=failureInputReadDsrv.slx  SimulationMode=Normal  VariantControl="strcmpi(vehicleParams.type, \"uuv_dsrv\")"  ModelReferenceVersion=1.1
  uuv_npsauv : ModelReference  ModelNameDialog=failureInputReadNpsAuv.slx  SimulationMode=Normal  VariantControl="strcmpi(vehicleParams.type, \"uuv_npsauv\")"  ModelReferenceVersion=1.1
  uuv_subsea : ModelReference  ModelNameDialog=failureInputReadUuvSubsea.slx  SimulationMode=Normal  VariantControl="strcmpi(vehicleParams.type, \"uuv_subsea\")"  ModelReferenceVersion=1.1
  vtol_tailsitter : ModelReference  DisableCoverage=on  ModelNameDialog=failureInputReadVtolTailsitter.slx  VariantControl="strcmpi(vehicleParams.type, \"vtol_tailsitter\")"  ModelReferenceVersion=1.6
  wheel_loader : ModelReference  ModelNameDialog=failureInputReadWheelLoader.slx  SimulationMode=Normal  VariantControl="strcmpi(vehicleParams.type, \"wheel_loader\")"  ModelReferenceVersion=1.1
  wheel_loader_simscape : ModelReference  ModelNameDialog=failureInputReadWheelLoaderSimscape.slx  SimulationMode=Normal  VariantControl="strcmpi(vehicleParams.type, \"wheel_loader_simscape\")"  ModelReferenceVersion=1.1
  FailureBus : Outport

== system VehicleSilSimulation/PX4 HITL Interface/Compute Timestamp ==
  Add : Sum
  Constant : Constant  Value=SampleTime*1e6  OutDataTypeStr=uint64  SampleTime=SampleTime
  Data Store Read : DataStoreRead  DataStoreName=Timestamp  SampleTime=SampleTime  IndexOptions=Index vector (dialog)  Indices=1  OutputSizes=1
  Data Store Write : DataStoreWrite  DataStoreName=Timestamp  SampleTime=SampleTime  IndexOptions=Index vector (dialog)  Indices=1  OutputSizes=1
  Timestamp : Outport
  wires:
  Data Store Read/1 -> Add/1
  Add/1 -> Timestamp/1, Data Store Write/1  "Timestamp"
  Constant/1 -> Add/2

== system VehicleSilSimulation/PX4 HITL Interface/HIL Sensor ==
  Acc : Inport
  Gyro : Inport  Port=2
  Mag : Inport  Port=3
  Pressure : Inport  Port=4
  Diff pressure : Inport  Port=5
  Time : Inport  Port=6
  HIL_SENSOR Creation subsystem : Subsystem
  MAVLink Serializer1 : uavmavlinklib/MAVLink Serializer  dialectSource=Select from standard MAVLink dialects  dialect=common.xml  dialectCustom=common.xml  version=2  messageType=HIL_SENSOR
  Rate Transition : RateTransition  OutPortSampleTime=SampleTime
  Terminator : Terminator
  HIL_SENSOR_bytes : Outport
  wires:
  Acc/1 -> HIL_SENSOR Creation subsystem/1(Acc)
  Gyro/1 -> HIL_SENSOR Creation subsystem/2(Gyro)
  Mag/1 -> HIL_SENSOR Creation subsystem/3(Mag)
  Pressure/1 -> HIL_SENSOR Creation subsystem/4(Pressure)
  Diff pressure/1 -> HIL_SENSOR Creation subsystem/5(Diff Pressure)
  Rate Transition/1 -> MAVLink Serializer1/1
  MAVLink Serializer1/2 -> Terminator/1
  MAVLink Serializer1/1 -> HIL_SENSOR_bytes/1
  HIL_SENSOR Creation subsystem/1(HIL Sensor) -> Rate Transition/1
  Time/1 -> HIL_SENSOR Creation subsystem/6(Time)

== system VehicleSilSimulation/PX4 HITL Interface/HIL_GPS ==
  LLA : Inport
  Velocity : Inport  Port=2
  GndSpeed : Inport  Port=3
  Course : Inport  Port=4
  Time : Inport  Port=5
  GPS : Subsystem
  GPS Serialization : Subsystem
  HIL_GPS_bytes : Outport
  wires:
  LLA/1 -> GPS Serialization/1(LLA)
  Velocity/1 -> GPS Serialization/2(Velocity)
  GndSpeed/1 -> GPS Serialization/3(GndSpeed)
  Course/1 -> GPS Serialization/4(Course)
  Time/1 -> GPS/2(Timestamp), GPS Serialization/5(Time)
  GPS Serialization/1(GPS Bytes) -> GPS/1(GPS Bytes)
  GPS/1(GPS Value) -> HIL_GPS_bytes/1
  GPS/2(Update GPS) -> GPS Serialization/Enable

== system VehicleSilSimulation/PX4 HITL Interface/Read actuator output ==
  From Autopilot : Inport
  Data Length : Inport  Port=2
  Constant : Constant  SampleTime=SampleTime
  Constant1 : Constant  Value=0  OutDataTypeStr=uint8  SampleTime=SampleTime
  Data Type Conversion : DataTypeConversion  OutDataTypeStr=double  SaturateOnIntegerOverflow=off  RndMeth=Floor
  Mux : Mux  Inputs=2
  Reshape : Reshape
  Selector : Selector  InputPortWidth=MAVLink_Input_Read_Size  IndexOptions=Starting and ending indices (port)  Indices=[1 3]  OutputSizes=1
  Switch : Switch  Criteria=u2 > Threshold  SaturateOnIntegerOverflow=off  InputSameDT=off
  Actuator_Bytes : Outport
  wires:
  Mux/1 -> Selector/2
  Constant/1 -> Mux/1
  Data Length/1 -> Data Type Conversion/1
  From Autopilot/1 -> Selector/1
  Switch/1 -> Reshape/1
  Selector/1 -> Switch/1
  Data Type Conversion/1 -> Switch/2, Mux/2
  Reshape/1 -> Actuator_Bytes/1
  Constant1/1 -> Switch/3

== system VehicleSilSimulation/PX4 HITL Interface/Send Heartbeat ==
  Timestamp : Inport
  GPS : Subsystem
  Heartbeat_Serialization : Subsystem
  Heartbeat Bytes : Outport
  wires:
  Heartbeat_Serialization/1(Heartbeat) -> GPS/1(Heartbeat Bytes)
  Timestamp/1 -> GPS/2(Timestamp)
  GPS/1(Update Heartbeat) -> Heartbeat_Serialization/Enable
  GPS/2(Heartbeat Value) -> Heartbeat Bytes/1

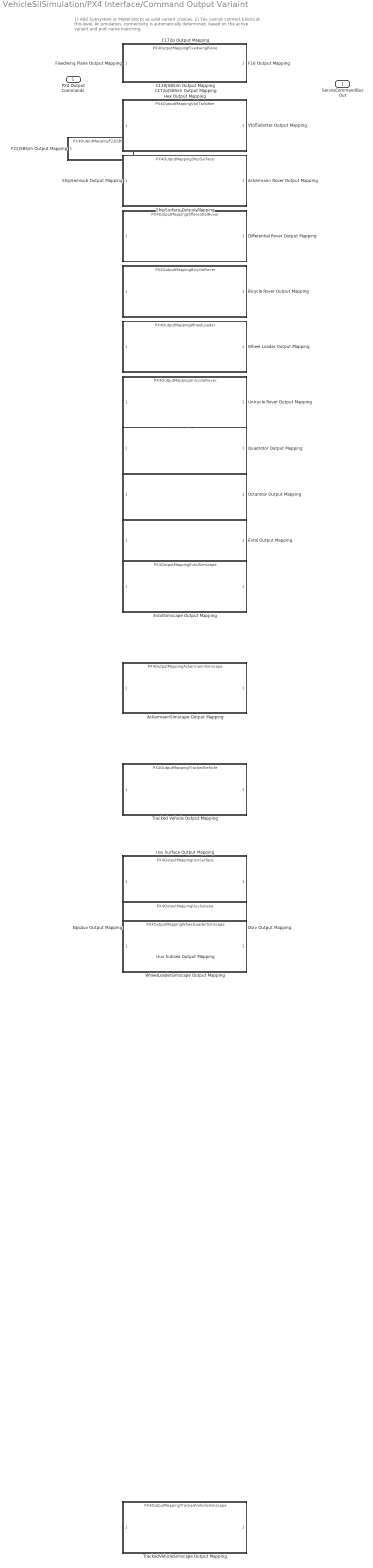
== system VehicleSilSimulation/PX4 Interface/Command Output Variaint ==
  note: 1) Add Subsystem or Model blocks as valid variant choices.
      | 2) You cannot connect blocks at this level. At simulation, connectivity is automatically
      | determined, based on the active variant and port name matching.
  PX4 Output Commands : Inport  PortDimensions=16
  Ackermann Rover Output Mapping : ModelReference  ModelNameDialog=PX4OutputMappingAckermannRover.slx  SimulationMode=Normal  VariantControl="strcmpi(vehicleParams.type, \"ackermann_rover\") & strcmpi(vehicleParams.controllerType, \"PX4\")"  ModelReferenceVersion=1.5
  AckermannSimscape Output Mapping : ModelReference  ModelNameDialog=PX4OutputMappingAckermannSimscape.slx  SimulationMode=Normal  VariantControl="strcmpi(vehicleParams.type, \"ackermann_simscape\") & strcmpi(vehicleParams.controllerType, \"PX4\")"  ModelReferenceVersion=1.5
  Bicycle Rover Output Mapping : ModelReference  ModelNameDialog=PX4OutputMappingBicycleRover.slx  SimulationMode=Normal  VariantControl="strcmpi(vehicleParams.type, \"bicycle_rover\") & strcmpi(vehicleParams.controllerType, \"PX4\")"  ModelReferenceVersion=1.1
  C130JSBSim Output Mapping : ModelReference  DisableCoverage=on  ModelNameDialog=PX4OutputMappingC130JSBSim  VariantControl="strcmpi(vehicleParams.type, \"c130JSBSim\") & strcmpi(vehicleParams.controllerType, \"PX4\")"  ModelReferenceVersion=5.0
  C172p Output Mapping : ModelReference  DisableCoverage=on  ModelNameDialog=PX4OutputMappingC172p  VariantControl="strcmpi(vehicleParams.type, \"c172p\") & strcmpi(vehicleParams.controllerType, \"PX4\")"  ModelReferenceVersion=5.0
  C172pJSBSim Output Mapping : ModelReference  DisableCoverage=on  ModelNameDialog=PX4OutputMappingC172pJSBSim.slx  VariantControl="strcmpi(vehicleParams.type, \"c172pJSBSim\") & strcmpi(vehicleParams.controllerType, \"PX4\")"  ModelReferenceVersion=5.0
  Differential Rover Output Mapping : ModelReference  ModelNameDialog=PX4OutputMappingDifferentialRover.slx  SimulationMode=Normal  VariantControl="strcmpi(vehicleParams.type, \"differential_rover\") & strcmpi(vehicleParams.controllerType, \"PX4\")"  ModelReferenceVersion=1.1
  Dsrv Output Mapping : ModelReference  ModelNameDialog=PX4OutputMappingDsrv.slx  SimulationMode=Normal  VariantControl="strcmpi(vehicleParams.type, \"uuv_dsrv\") & strcmpi(vehicleParams.controllerType, \"PX4\")"  ModelReferenceVersion=1.1
  Evtol Output Mapping : ModelReference  ModelNameDialog=PX4OutputMappingEvtol.slx  SimulationMode=Normal  VariantControl="strcmpi(vehicleParams.type, \"evtol\") & strcmpi(vehicleParams.controllerType, \"PX4\")"  ModelReferenceVersion=5.0
  EvtolSimscape Output Mapping : ModelReference  ModelNameDialog=PX4OutputMappingEvtolSimscape.slx  SimulationMode=Normal  VariantControl="strcmpi(vehicleParams.type, \"evtol_simscape\") & strcmpi(vehicleParams.controllerType, \"PX4\")"  ModelReferenceVersion=5.0
  F16 Output Mapping : ModelReference  DisableCoverage=on  ModelNameDialog=PX4OutputMappingF16.slx  VariantControl="strcmpi(vehicleParams.type, \"F16\") & strcmpi(vehicleParams.controllerType, \"PX4\")"  ModelReferenceVersion=1.8
  F22JSBSim Output Mapping : ModelReference  ModelNameDialog=PX4OutputMappingF22JSBSim  SimulationMode=Normal  VariantControl="strcmpi(vehicleParams.type, \"f22JSBSim\") & strcmpi(vehicleParams.controllerType, \"PX4\")"  ModelReferenceVersion=5.0
  Fixedwing Plane Output Mapping : ModelReference  DisableCoverage=on  ModelNameDialog=PX4OutputMappingFixedwingPlane.slx  VariantControl="strcmpi(vehicleParams.type, \"fixedwing_plane\") & strcmpi(vehicleParams.controllerType, \"PX4\")"  ModelReferenceVersion=5.0
  Hex Output Mapping : ModelReference  ModelNameDialog=PX4OutputMappingHex.slx  VariantControl="strcmpi(vehicleParams.type, \"hexarotor\") & strcmpi(vehicleParams.controllerType, \"PX4\")"  ModelReferenceVersion=1.15
  NpsAuv Output Mapping : ModelReference  ModelNameDialog=PX4OutputMappingNpsAuv.slx  SimulationMode=Normal  VariantControl="strcmpi(vehicleParams.type, \"uuv_npsauv\") & strcmpi(vehicleParams.controllerType, \"PX4\")"  ModelReferenceVersion=1.1
  Octarotor Output Mapping : ModelReference  ModelNameDialog=PX4OutputMappingOctarotor.slx  SimulationMode=Normal  VariantControl="strcmpi(vehicleParams.type, \"octarotor\") & strcmpi(vehicleParams.controllerType, \"PX4\")"  ModelReferenceVersion=1.1
  Quadrotor Output Mapping : ModelReference  ModelNameDialog=PX4OutputMappingQuadrotor.slx  SimulationMode=Normal  VariantControl="strcmpi(vehicleParams.type, \"quadrotor\") & strcmpi(vehicleParams.controllerType, \"PX4\")"  ModelReferenceVersion=1.1
  ShipSemisub Output Mapping : ModelReference  ModelNameDialog=PX4OutputMappingShipSemisub.slx  SimulationMode=Normal  VariantControl="strcmpi(vehicleParams.type, \"ship_semisub\") & strcmpi(vehicleParams.controllerType, \"PX4\")"  ModelReferenceVersion=1.6
  ShipSurface Output Mapping : ModelReference  ModelNameDialog=PX4OutputMappingShipSurface.slx  SimulationMode=Normal  VariantControl="strcmpi(vehicleParams.type, \"ship_surface\") & strcmpi(vehicleParams.controllerType, \"PX4\")"  ModelReferenceVersion=1.6
  Tracked Vehicle Output Mapping : ModelReference  ModelNameDialog=PX4OutputMappingTrackedVehicle.slx  SimulationMode=Normal  VariantControl="strcmpi(vehicleParams.type, \"tracked_vehicle\") & strcmpi(vehicleParams.controllerType, \"PX4\")"  ModelReferenceVersion=1.1
  TrackedVehicleSimscape Output Mapping : ModelReference  ModelNameDialog=PX4OutputMappingTrackedVehicleSimscape.slx  SimulationMode=Normal  VariantControl="strcmpi(vehicleParams.type, \"tracked_vehicle_simscape\") & strcmpi(vehicleParams.controllerType, \"PX4\")"  ModelReferenceVersion=1.1
  Unicycle Rover Output Mapping : ModelReference  ModelNameDialog=PX4OutputMappingUnicycleRover.slx  SimulationMode=Normal  VariantControl="strcmpi(vehicleParams.type, \"unicycle_rover\") & strcmpi(vehicleParams.controllerType, \"PX4\")"  ModelReferenceVersion=1.1
  Usv Surface Output Mapping : ModelReference  ModelNameDialog=PX4OutputMappingUsvSurface.slx  SimulationMode=Normal  VariantControl="strcmpi(vehicleParams.type, \"usv_surface\") & strcmpi(vehicleParams.controllerType, \"PX4\")"  ModelReferenceVersion=1.1
  Uuv Subsea Output Mapping : ModelReference  ModelNameDialog=PX4OutputMappingUuvSubsea.slx  SimulationMode=Normal  VariantControl="strcmpi(vehicleParams.type, \"uuv_subsea\") & strcmpi(vehicleParams.controllerType, \"PX4\")"  ModelReferenceVersion=1.1
  VtolTailsitter Output Mapping : ModelReference  ModelNameDialog=PX4OutputMappingVtolTailsitter.slx  VariantControl="strcmpi(vehicleParams.type, \"vtol_tailsitter\") & strcmpi(vehicleParams.controllerType, \"PX4\")"  ModelReferenceVersion=1.5
  Wheel Loader Output Mapping : ModelReference  ModelNameDialog=PX4OutputMappingWheelLoader.slx  SimulationMode=Normal  VariantControl="strcmpi(vehicleParams.type, \"wheel_loader\") & strcmpi(vehicleParams.controllerType, \"PX4\")"  ModelReferenceVersion=1.1
  WheelLoaderSimscape Output Mapping : ModelReference  ModelNameDialog=PX4OutputMappingWheelLoaderSimscape.slx  SimulationMode=Normal  VariantControl="strcmpi(vehicleParams.type, \"wheel_loader_simscape\") & strcmpi(vehicleParams.controllerType, \"PX4\")"  ModelReferenceVersion=1.1
  ServosCommandBusOut : Outport  OutDataTypeStr=Bus: ServosCommandBus

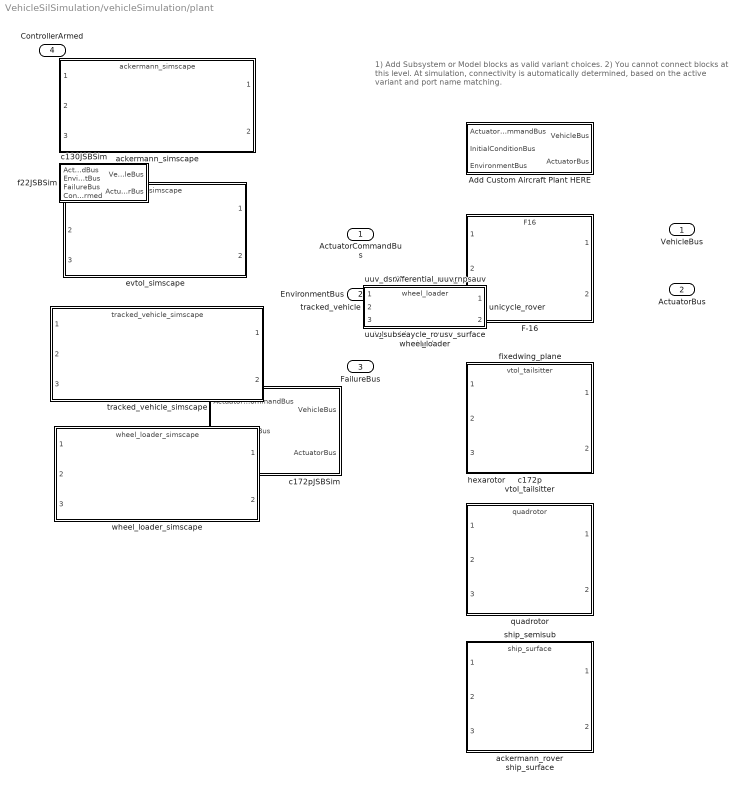
== system VehicleSilSimulation/vehicleSimulation/plant ==
  note: 1) Add Subsystem or Model blocks as valid variant choices.
      | 2) You cannot connect blocks at this level. At simulation, connectivity is automatically
      | determined, based on the active variant and port name matching.
  ActuatorCommandBus : Inport  OutDataTypeStr=Bus: ActuatorCommandBus  LockScale=on
  EnvironmentBus : Inport  Port=2  OutDataTypeStr=Bus: EnvironmentBus
  FailureBus : Inport  Port=3  OutDataTypeStr=Bus: FailureBus
  ControllerArmed : Inport  Port=4
  Add Custom Aircraft Plant HERE : Subsystem  VariantControl="strcmpi(vehicleParams.type ,\"Custom\")"
  F-16 : ModelReference  ModelNameDialog=F16.slx  VariantControl="strcmpi(vehicleParams.baseVehicleType ,\"F-16\")"  ModelReferenceVersion=1.120
  ackermann_rover : ModelReference  ModelNameDialog=ackermann_rover  SimulationMode=Normal  VariantControl="strcmpi(vehicleParams.type ,\"ackermann_rover\")"  ModelReferenceVersion=5.1
  ackermann_simscape : ModelReference  ModelNameDialog=ackermann_simscape  VariantControl="strcmpi(vehicleParams.type ,\"ackermann_simscape\")"  ModelReferenceVersion=5.1
  bicycle_rover : ModelReference  ModelNameDialog=bicycle_rover  SimulationMode=Normal  VariantControl="strcmpi(vehicleParams.type ,\"bicycle_rover\")"  ModelReferenceVersion=5.0
  c130JSBSim : Subsystem  VariantControl="strcmpi(vehicleParams.type ,\"c130JSBSim\")"
  c172p : ModelReference  ModelNameDialog=c172p  SimulationMode=Normal  VariantControl="strcmpi(vehicleParams.type ,\"c172p\")"  ModelReferenceVersion=5.0
  c172pJSBSim : Subsystem  VariantControl="strcmpi(vehicleParams.type ,\"c172pJSBSim\")"
  differential_rover : ModelReference  ModelNameDialog=differential_rover  SimulationMode=Normal  VariantControl="strcmpi(vehicleParams.type ,\"differential_rover\")"  ModelReferenceVersion=5.0
  evtol : ModelReference  ModelNameDialog=evtol  SimulationMode=Normal  VariantControl="strcmpi(vehicleParams.type ,\"evtol\")"  ModelReferenceVersion=1.56
  evtol_simscape : ModelReference  ModelNameDialog=evtol_simscape  VariantControl="strcmpi(vehicleParams.type ,\"evtol_simscape\")"  ModelReferenceVersion=5.1
  f22JSBSim : Subsystem  VariantControl="strcmpi(vehicleParams.type ,\"f22JSBSim\")"
  fixedwing_plane : ModelReference  ModelNameDialog=fixedwing_plane.slx  SimulationMode=Normal  VariantControl="strcmpi(vehicleParams.type ,\"fixedwing_plane\")"  ModelReferenceVersion=5.0
  hexarotor : ModelReference  ModelNameDialog=hexarotor.slx  SimulationMode=Normal  VariantControl="strcmpi(vehicleParams.type ,\"hexarotor\")"  ModelReferenceVersion=1.56
  octarotor : ModelReference  ModelNameDialog=octarotor  SimulationMode=Normal  VariantControl="strcmpi(vehicleParams.type ,\"octarotor\")"  ModelReferenceVersion=1.56
  quadrotor : ModelReference  ModelNameDialog=quadrotor  SimulationMode=Normal  VariantControl="strcmpi(vehicleParams.type ,\"quadrotor\")"  ModelReferenceVersion=1.56
  ship_semisub : ModelReference  ModelNameDialog=ship_semisub.slx  SimulationMode=Normal  VariantControl="strcmpi(vehicleParams.type ,\"ship_semisub\")"  ModelReferenceVersion=5.4
  ship_surface : ModelReference  ModelNameDialog=ship_surface.slx  SimulationMode=Normal  VariantControl="strcmpi(vehicleParams.type ,\"ship_surface\")"  ModelReferenceVersion=5.3
  tracked_vehicle : ModelReference  ModelNameDialog=tracked_vehicle  SimulationMode=Normal  VariantControl="strcmpi(vehicleParams.type ,\"tracked_vehicle\")"  ModelReferenceVersion=5.1
  tracked_vehicle_simscape : ModelReference  ModelNameDialog=tracked_vehicle_simscape  VariantControl="strcmpi(vehicleParams.type ,\"tracked_vehicle_simscape\")"  ModelReferenceVersion=5.1
  unicycle_rover : ModelReference  ModelNameDialog=unicycle_rover  SimulationMode=Normal  VariantControl="strcmpi(vehicleParams.type ,\"unicycle_rover\")"  ModelReferenceVersion=5.0
  usv_surface : ModelReference  ModelNameDialog=usv_surface  SimulationMode=Normal  VariantControl="strcmpi(vehicleParams.type ,\"usv_surface\")"  ModelReferenceVersion=5.2
  uuv_dsrv : ModelReference  ModelNameDialog=uuv_dsrv.slx  SimulationMode=Normal  VariantControl="strcmpi(vehicleParams.type ,\"uuv_dsrv\")"  ModelReferenceVersion=5.3
  uuv_npsauv : ModelReference  ModelNameDialog=uuv_npsauv.slx  SimulationMode=Normal  VariantControl="strcmpi(vehicleParams.type ,\"uuv_npsauv\")"  ModelReferenceVersion=5.3
  uuv_subsea : ModelReference  ModelNameDialog=uuv_subsea  SimulationMode=Normal  VariantControl="strcmpi(vehicleParams.type ,\"uuv_subsea\")"  ModelReferenceVersion=5.2
  vtol_tailsitter : ModelReference  ModelNameDialog=vtol_tailsitter.slx  SimulationMode=Normal  VariantControl="strcmpi(vehicleParams.type ,\"vtol_tailsitter\")"  ModelReferenceVersion=1.56
  wheel_loader : ModelReference  ModelNameDialog=wheel_loader  SimulationMode=Normal  VariantControl="strcmpi(vehicleParams.type ,\"wheel_loader\")"  ModelReferenceVersion=5.0
  wheel_loader_simscape : ModelReference  ModelNameDialog=wheel_loader_simscape  VariantControl="strcmpi(vehicleParams.type ,\"wheel_loader_simscape\")"  ModelReferenceVersion=5.0
  VehicleBus : Outport
  ActuatorBus : Outport  Port=2

== system VehicleSilSimulation/visualizationVariant/FlightGearVisualizationF16 ==
  note: Visualization
  VehicleBus : Inport
  FlightGear Preconfigured 6DoF Animation : aerolibfltsims/FlightGear Preconfigured 6DoF Animation  xFlightGearVersion=v2019.1  DestinationIpAddress=127.0.0.1  DestinationPort=5502  SampleTime=-1  packetVersion=24
  Motion Conversion for Animation : Subsystem
      mask Display:
      | port_label('input',1,'ACBus')
      | port_label('output',1,'\lambda,L,h,\phi,\theta,\psi','texmode','on')
  Terminator : Terminator
  Terminator1 : Terminator
  wires:
  Motion Conversion for Animation/1(FGInterface) -> FlightGear Preconfigured 6DoF Animation/1
  VehicleBus/1 -> Motion Conversion for Animation/1(VehicleBus)
  Motion Conversion for Animation/2(XYZ_NED) -> Terminator/1
  Motion Conversion for Animation/3(AttitudeQuaternion) -> Terminator1/1

== system VehicleSilSimulation/visualizationVariant/FlightGearVisualizationFixedWing ==
  VehicleBus : Inport
  FlightGear Preconfigured 6DoF Animation : aerolibfltsims/FlightGear Preconfigured 6DoF Animation  xFlightGearVersion=v2019.1  DestinationIpAddress=127.0.0.1  DestinationPort=5502  SampleTime=-1  packetVersion=24
  Motion Conversion for Animation : Subsystem
      mask Display:
      | port_label('input',1,'ACBus')
      | port_label('output',1,'\lambda,L,h,\phi,\theta,\psi','texmode','on')
  Terminator : Terminator
  Terminator1 : Terminator
  wires:
  VehicleBus/1 -> Motion Conversion for Animation/1(VehicleBus)
  Motion Conversion for Animation/1(FGInterface) -> FlightGear Preconfigured 6DoF Animation/1
  Motion Conversion for Animation/2(XYZ_NED) -> Terminator/1
  Motion Conversion for Animation/3(AttitudeQuaternion) -> Terminator1/1
